simulink model "Prop_VarCoefPoly1"  (R2016b)
settings: Solver=VariableStepAuto  StartTime=0.0  StopTime=10.0  RelTol=1e-3
undefined symbols (not defined in the file or in its folder): AC
libraries: OpenFlightUtilLib x6
settings Model: Creator=rega0051  LastModifiedBy=rega0051
settings DataIOCC: SaveOutput=off  SignalLogging=off  DSMLogging=off  SaveTime=off

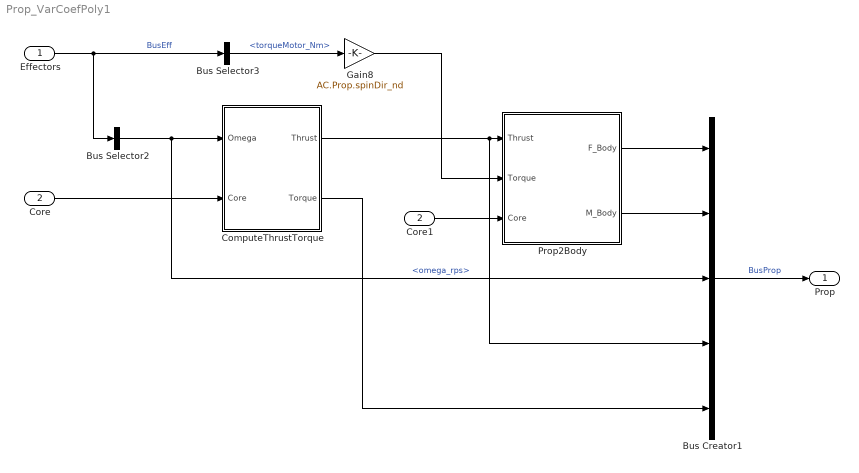
== system Prop_VarCoefPoly1 ==
  Effectors : Inport  OutDataTypeStr=Bus: BusEff  SampleTime=0
      settings: AttributesFormatString=%<OutDataTypeStr>
  Core : Inport  Port=2  OutDataTypeStr=Bus: BusCore
      settings: AttributesFormatString=%<OutDataTypeStr>
  Bus Selector2 : BusSelector  OutputSignals=BusMotor.omega_rps
  Bus Selector3 : BusSelector  OutputSignals=BusMotor.torqueMotor_Nm
  Bus Creator1 : BusCreator  Inputs=5  OutDataTypeStr=Bus: BusProp  NonVirtualBus=on
      settings: AttributesFormatString=%<OutDataTypeStr>  InheritFromInputs=off
  ComputeThrustTorque : Subsystem
  Core1 : InportShadow  Port=2  OutDataTypeStr=Bus: BusCore
      settings: AttributesFormatString=%<OutDataTypeStr>
  Gain8 : Gain  Gain=AC.Prop.spinDir_nd  SaturateOnIntegerOverflow=on  OutDataTypeStr=Inherit: Same as input  ParamDataTypeStr=Inherit: Same as input
      settings: AttributesFormatString=%<Gain>
  Prop2Body : Subsystem
  Prop : Outport  OutDataTypeStr=Bus: BusProp  SampleTime=0
      settings: AttributesFormatString=%<OutDataTypeStr>
  wires:
  Core/1 -> ComputeThrustTorque/2(Core)
  Prop2Body/2(M_Body) -> Bus Creator1/2
  ComputeThrustTorque/1(Thrust) -> Prop2Body/1(Thrust), Bus Creator1/4
  Prop2Body/1(F_Body) -> Bus Creator1/1
  Core1/1 -> Prop2Body/3(Core)
  Bus Creator1/1 -> Prop/1  "BusProp"
  Gain8/1 -> Prop2Body/2(Torque)
  Bus Selector2/1 -> Bus Creator1/3, ComputeThrustTorque/1(Omega)  "<omega_rps>"
  Effectors/1 -> Bus Selector3/1, Bus Selector2/1  "BusEff"
  Bus Selector3/1 -> Gain8/1  "<torqueMotor_Nm>"
  ComputeThrustTorque/2(Torque) -> Bus Creator1/5

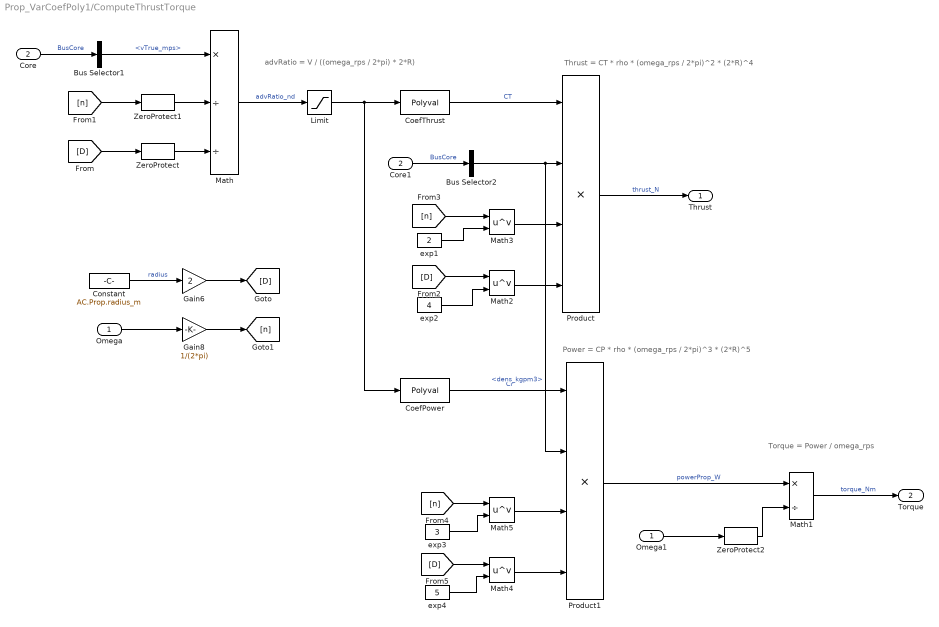
== system Prop_VarCoefPoly1/ComputeThrustTorque ==
  note: Power = CP * rho * (omega_rps / 2*pi)^3 * (2*R)^5
  note: Thrust = CT * rho * (omega_rps / 2*pi)^2 * (2*R)^4
  note: advRatio = V / ((omega_rps / 2*pi) * 2*R)
  note: Torque = Power / omega_rps
  Omega : Inport  OutDataTypeStr=double
  Core : Inport  Port=2  OutDataTypeStr=double
  Bus Selector1 : BusSelector  OutputSignals=BusAux.BusFlow.vTrue_mps
  Bus Selector2 : BusSelector  OutputSignals=BusEnv.BusAtmos.dens_kgpm3
  CoefPower : Polyval  Coefs=AC.Prop.CP
      settings: AttributesFormatString=%<Coefs>
  CoefThrust : Polyval  Coefs=AC.Prop.CT
      settings: AttributesFormatString=%<Coefs>
  Constant : Constant  Value=AC.Prop.radius_m
      settings: AttributesFormatString=%<Value>
  Core1 : InportShadow  Port=2  OutDataTypeStr=double
  Gain6 : Gain  Gain=2  SaturateOnIntegerOverflow=on  OutDataTypeStr=Inherit: Same as input  ParamDataTypeStr=Inherit: Same as input
  Gain8 : Gain  Gain=1/(2*pi)  SaturateOnIntegerOverflow=on  OutDataTypeStr=Inherit: Same as input  ParamDataTypeStr=Inherit: Same as input
      settings: AttributesFormatString=%<Gain>
  Limit : Saturate  UpperLimit=0.7  LowerLimit=0
  Math : Product  Inputs=*//  SaturateOnIntegerOverflow=on  InputSameDT=on  OutDataTypeStr=Inherit: Same as first input
  Math1 : Product  Inputs=*/  SaturateOnIntegerOverflow=on  InputSameDT=on  OutDataTypeStr=Inherit: Same as first input
  Math{2..5} (4 alike) : Math  Operator=pow  SaturateOnIntegerOverflow=on
  Omega1 : InportShadow  OutDataTypeStr=double
  Product : Product  Inputs=4  SaturateOnIntegerOverflow=on  InputSameDT=on  OutDataTypeStr=Inherit: Same as first input
  Product1 : Product  Inputs=4  SaturateOnIntegerOverflow=on  InputSameDT=on  OutDataTypeStr=Inherit: Same as first input
  ZeroProtect : OpenFlightUtilLib/Math/ZeroProtect  epsilon=eps
  ZeroProtect1 : OpenFlightUtilLib/Math/ZeroProtect  epsilon=eps
  ZeroProtect2 : OpenFlightUtilLib/Math/ZeroProtect  epsilon=eps
  exp1 : Constant  Value=2
  exp2 : Constant  Value=4
  exp3 : Constant  Value=3
  exp4 : Constant  Value=5
  Thrust : Outport
  Torque : Outport  Port=2
  wires:
  Math1/1 -> Torque/1  "torque_Nm"
  ZeroProtect2/1 -> Math1/2
  Omega1/1 -> ZeroProtect2/1
  ZeroProtect1/1 -> Math/2
  ZeroProtect/1 -> Math/3
  [D] -> ZeroProtect/1
  [n] -> ZeroProtect1/1
  Gain8/1 -> [n]
  Omega/1 -> Gain8/1
  Constant/1 -> Gain6/1  "radius"
  Gain6/1 -> [D]
  CoefPower/1 -> Product1/1  "CP"
  exp3/1 -> Math5/2
  [D] -> Math4/1
  [n] -> Math5/1
  Math5/1 -> Product1/3
  exp4/1 -> Math4/2
  Math4/1 -> Product1/4
  exp1/1 -> Math3/2
  [D] -> Math2/1
  [n] -> Math3/1
  Limit/1 -> CoefPower/1, CoefThrust/1
  Product1/1 -> Math1/1  "powerProp_W"
  Math/1 -> Limit/1  "advRatio_nd"
  Math3/1 -> Product/3
  exp2/1 -> Math2/2
  Math2/1 -> Product/4
  Product/1 -> Thrust/1  "thrust_N"
  CoefThrust/1 -> Product/1  "CT"
  Core/1 -> Bus Selector1/1  "BusCore"
  Bus Selector1/1 -> Math/1  "<vTrue_mps>"
  Bus Selector2/1 -> Product1/2, Product/2  "<dens_kgpm3>"
  Core1/1 -> Bus Selector2/1  "BusCore"

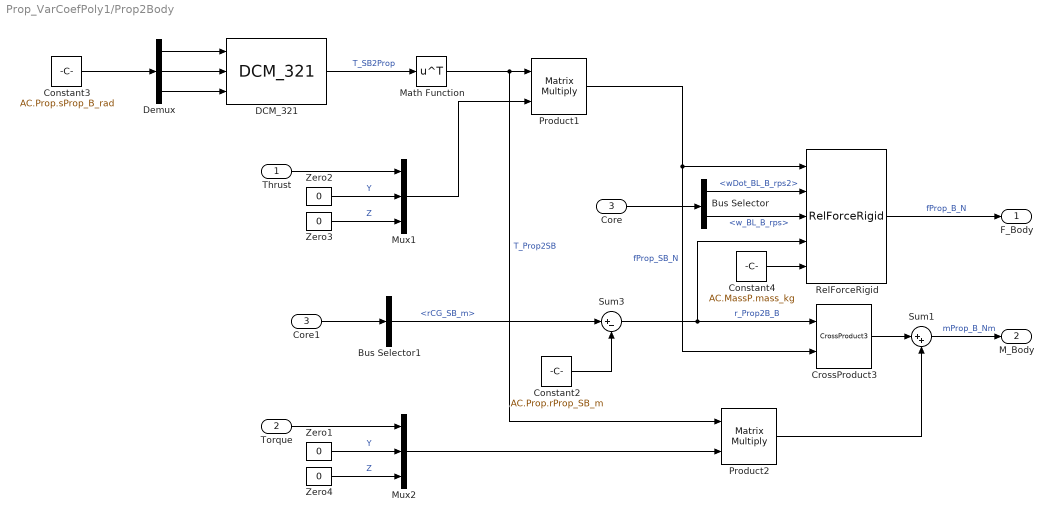
== system Prop_VarCoefPoly1/Prop2Body ==
  Thrust : Inport
  Torque : Inport  Port=2
  Core : Inport  Port=3
  Bus Selector : BusSelector  OutputSignals=BusEom.wDot_BL_B_rps2,BusEom.w_BL_B_rps
  Bus Selector1 : BusSelector  OutputSignals=BusEom.rCG_SB_m
  Constant2 : Constant  Value=AC.Prop.rProp_SB_m
      settings: AttributesFormatString=%<Value>
  Constant3 : Constant  Value=AC.Prop.sProp_B_rad
      settings: AttributesFormatString=%<Value>
  Constant4 : Constant  Value=AC.MassP.mass_kg
      settings: AttributesFormatString=%<Value>
  Core1 : InportShadow  Port=3
  CrossProduct3 : OpenFlightUtilLib/Math/CrossProduct3
  DCM_321 : OpenFlightUtilLib/Transformations/DCM_321
  Demux : Demux  Outputs=3
  Math Function : Math  Operator=transpose  SaturateOnIntegerOverflow=on
  Mux1 : Mux  Inputs=3
  Mux2 : Mux  Inputs=3
  Product1 : Product  Multiplication=Matrix(*)  RndMeth=Zero
  Product2 : Product  Multiplication=Matrix(*)  RndMeth=Zero
  RelForceRigid : OpenFlightUtilLib/Kinematics and Dynamics/RelForceRigid
  Sum1 : Sum  Inputs=|++  SaturateOnIntegerOverflow=on
  Sum3 : Sum  Inputs=|+-  SaturateOnIntegerOverflow=on
  Zero{1..4} (4 alike) : Constant  Value=0
  F_Body : Outport
  M_Body : Outport  Port=2
  wires:
  Core1/1 -> Bus Selector1/1
  Mux2/1 -> Product2/2
  Torque/1 -> Mux2/1
  Zero1/1 -> Mux2/2  "Y"
  Zero4/1 -> Mux2/3  "Z"
  Mux1/1 -> Product1/2
  Zero2/1 -> Mux1/2  "Y"
  Zero3/1 -> Mux1/3  "Z"
  Constant4/1 -> RelForceRigid/5
  Product2/1 -> Sum1/2
  DCM_321/1 -> Math Function/1  "T_SB2Prop"
  Demux/2 -> DCM_321/2
  Demux/1 -> DCM_321/1
  Demux/3 -> DCM_321/3
  Constant3/1 -> Demux/1
  Sum1/1 -> M_Body/1  "mProp_B_Nm"
  CrossProduct3/1 -> Sum1/1
  RelForceRigid/1 -> F_Body/1  "fProp_B_N"
  Core/1 -> Bus Selector/1
  Sum3/1 -> RelForceRigid/4, CrossProduct3/1  "r_Prop2B_B"
  Product1/1 -> CrossProduct3/2, RelForceRigid/1  "fProp_SB_N"
  Math Function/1 -> Product1/1, Product2/1  "T_Prop2SB"
  Thrust/1 -> Mux1/1
  Bus Selector/2 -> RelForceRigid/3  "<w_BL_B_rps>"
  Bus Selector/1 -> RelForceRigid/2  "<wDot_BL_B_rps2>"
  Constant2/1 -> Sum3/2
  Bus Selector1/1 -> Sum3/1  "<rCG_SB_m>"
